simulink model "reg"  (R2024b)
settings: Solver=VariableStepAuto  StartTime=tspan(1)  StopTime=tspan(2)  RelTol=1e-3
values from neighbouring files (symbols this model uses):
  den = conv([T1 1], [1 0])    [motor.m]
  desr = [35 40]    [motor.m]
  desr_val = 0.01    [motor.m]
  num = K1    (= 100)    [motor.m]
  Reg = GhReg    [motor.m]
  step_t = 5    [motor.m]
  u_des = 1    [motor.m]
settings Model: Creator=markminerov  LastModifiedBy=markminerov

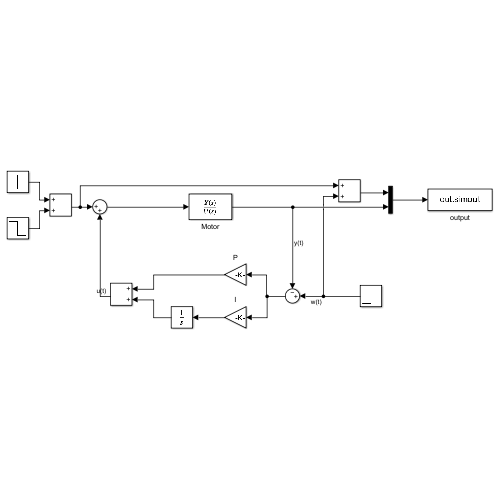
[thumbnail: Simulink's stored preview of the top-level diagram]
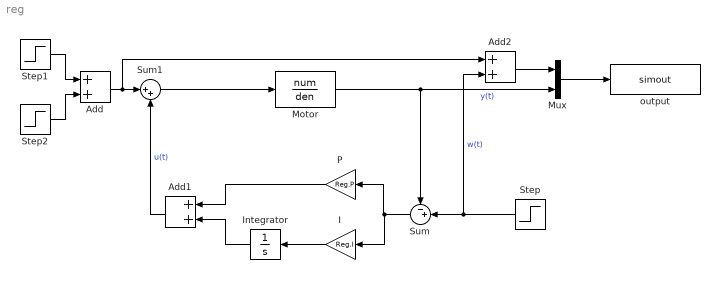
== system reg ==
  Add : Sum
  Add1 : Sum
  Add2 : Sum
  I : Gain  Gain=Reg.I
  Integrator : Integrator
  Motor : TransferFcn  Numerator=num  Denominator=den
  Mux : Mux  Inputs=2
  P : Gain  Gain=Reg.P
  Step : Step  Time=step_t  After=u_des  SampleTime=0
  Step1 : Step  Time=desr(2)  After=desr_val  SampleTime=0
  Step2 : Step  Time=desr(1)  After=-desr_val  SampleTime=0
  Sum : Sum  Inputs=-+|
  Sum1 : Sum  Inputs=|++
  output : ToWorkspace  VariableName=simout  SaveFormat=Timeseries  SampleTime=-1
  wires:
  I/1 -> Integrator/1
  Integrator/1 -> Add1/2
  P/1 -> Add1/1
  Add1/1 -> Sum1/2  "u(t)"
  Motor/1 -> Sum/1, Mux/2  "y(t)"
  Step/1 -> Sum/2, Add2/2  "w(t)"
  Sum/1 -> I/1, P/1
  Mux/1 -> output/1
  Step1/1 -> Add/1
  Step2/1 -> Add/2
  Add/1 -> Add2/1, Sum1/1
  Sum1/1 -> Motor/1
  Add2/1 -> Mux/1
